simulink model "Model"  (R2021b)
settings: Solver=FixedStepAuto  StartTime=0.0  StopTime=T  FixedStep=0.1  RelTol=1e-3
values from neighbouring files (symbols this model uses):
  A = zeros(length(w_0))    [Model_script.m]
  a = R_E + 550    [Model_script.m]    (also in Orbit_Model.m)
  A0 = eye(3)    [Model_script.m]
  actuators_matrix = [1 0 0; 0 1 0; 0 0 1]    [Model_script.m]
  alpha = deg2rad(11.5)    [Model_script.m]
  Area_mb = diag([A1 A2 A3 A4 A5 A6])    [Model_script.m]
  Area_sp = diag([A7 A8 A9 A10])    [Model_script.m]
  around_boresight = deg2rad(dms2degrees([0,0,around_boresight]))    [Model_script.m]
  B = diag([1/Ix, 1/Iy, 1/Iz])    [Model_script.m]
  cross_boresight = deg2rad(dms2degrees([0,0,cross_boresight]))    [Model_script.m]
  e = 0.0001824    [Model_script.m]    (also in Orbit_Model.m)
  epsilon = deg2rad(23.45)    [Model_script.m]
  H0 = ( g1_0^2 + g1_1^2 + h1_1^2 )^(1/2)    (= 3.0115258674e-05)    [Model_script.m]
  h_N_target = [0; 0; I(3,3)*n]    [Model_script.m]
  I = I_mb + I_depl    [Model_script.m]
  i = deg2rad(53.0545)    [Model_script.m]    (also in Orbit_Model.m)
  I_inv = inv(I)    [Model_script.m]
  i_matrix = [1 0 0; 0 cos(i) sin(i); 0 -sin(i) cos(i)]    [Model_script.m]
  Kb = 1e10    (= 10000000000)    [Model_script.m]
  Kd = 5*1e-4*ones(length(w_0),1)    [Model_script.m]
  Kp = 5*1e-3*ones(length(w_0),1)    [Model_script.m]
  m = [0.01; 0.05; 0.01]    [Model_script.m]
  m_N_unit = zeros(size(m_N,1),size(m_N,2))    [Model_script.m]
  mu_E = astroConstants(13)    [Model_script.m]    (also in Orbit_Model.m)
  n = sqrt(mu_E/(a^3))    [Model_script.m]    (also in Orbit_Model.m)
  n4 = -n1    [Model_script.m]
  N_b_mb = [n1'; n2'; n3'; n4'; n5'; n6']    [Model_script.m]
  N_b_sp = [n7'; n8'; n9'; n10']    [Model_script.m]
  n_sun = 2*pi/T_sun    (= 1.99238499086e-07)    [Model_script.m]
  P = Fe/c    (= 4.52666666667e-06)    [Model_script.m]
  Q = zeros(length(w_0))    [Model_script.m]
  R = zeros(length(w_0))    [Model_script.m]
  R_E = astroConstants(23)    [Model_script.m]    (also in Orbit_Model.m)
  r_mb = [base/2 0 0; 0 base/2 0; 0 0 height/2; -base/2 0 0; 0 -base/2 0; 0 0 -height/2]    [Model_script.m]
  r_sp = [0 length_p1/2+base/2 0; 0 length_p1/2+base/2 0; 0 -length_p2/2-base/2 0; 0 -length_p2/2-base/2 0]    [Model_script.m]
  rho_s_mb = 0.3    [Model_script.m]
  rho_s_sp = 0    [Model_script.m]
  Rs = astroConstants(2)    [Model_script.m]
  star_sensor_tolerance = deg2rad(star_sensor_tolerance)    [Model_script.m]
  theta0 = deg2rad(0)    [Model_script.m]    (also in Orbit_Model.m)
  unit = [1 0 0]'    [Model_script.m]
  v1 = [0 1 -1]'    [Model_script.m]
  v2 = [-1 0 1]'    [Model_script.m]
  v3 = [1 -1 0]'    [Model_script.m]
  w_0 = [wx_0 wy_0 wz_0]'    [Model_script.m]
  w_E = deg2rad(15.04)/3600    [Model_script.m]    (also in Orbit_Model.m = deg2rad(15.04/3600))
  w_target = [0; 0; n]    [Model_script.m]
  weight = 1/6    (= 0.166666666667)    [Model_script.m]
  wy_0 = 0.7    [Model_script.m]
undefined symbols (not defined in the file or in its folder): phi0, psi0, q0
libraries: matrix_library x15, vrlib x12, dspmtrx3 x3, sharedutil x2
(part 2 of 2)

== system Model/Environment/GG Torque/Gravity Gradient ==
  A_BL : Inport
  R_orbit : Inport  Port=2
  Constant4 : Constant  Value=I
  Cross Product1 : matrix_library/Cross Product
      settings: SourceProductBaseCode=SL
  MatrixMultiply4 : Product  Multiplication=Matrix(*)
  Product : Product
  To Workspace : ToWorkspace  VariableName=c_vector  SampleTime=-1
  creation of coefficient 3*mu_E/(R^3) : Subsystem
  creation of vector c : Subsystem
  T_GG : Outport
  wires:
  Constant4/1 -> MatrixMultiply4/1
  MatrixMultiply4/1 -> Cross Product1/2
  Cross Product1/1 -> Product/2
  Product/1 -> T_GG/1
  creation of vector c/1(c) -> To Workspace/1, MatrixMultiply4/2, Cross Product1/1
  A_BL/1 -> creation of vector c/1(A_BL)
  R_orbit/1 -> creation of coefficient 3*mu_E/(R^3)/1(In1)
  creation of coefficient 3*mu_E/(R^3)/1(Out1) -> Product/1

== system Model/Environment/GG Torque/Transformation from A_B//N to A_B//L ==
  A_B/N : Inport
  theta : Inport  Port=2
  Constant : Constant  Value=i_matrix
  Matrix Multiply : Product  Multiplication=Matrix(*)
  MatrixMultiply1 : Product  Multiplication=Matrix(*)
  Transpose : Math  Operator=transpose  SaturateOnIntegerOverflow=on
  creation of A L/N : Subsystem
  A_B/L : Outport
  wires:
  A_B/N/1 -> MatrixMultiply1/1
  Transpose/1 -> MatrixMultiply1/2
  MatrixMultiply1/1 -> A_B/L/1  "A_BL"
  creation of A L/N/1(A_L/N) -> Matrix Multiply/1
  Constant/1 -> Matrix Multiply/2
  Matrix Multiply/1 -> Transpose/1
  theta/1 -> creation of A L/N/1(theta)

== system Model/Environment/Magnetic Torque/magnetic field of Earth (modelled as dipole) in body frame ==
  A_B/N : Inport
  r_N : Inport  Port=2
  Matrix Multiply : Product  Multiplication=Matrix(*)
  b_N : Subsystem
  b_B : Outport
  wires:
  b_N/1(b_N) -> Matrix Multiply/2
  r_N/1 -> b_N/1(r_N)
  A_B/N/1 -> Matrix Multiply/1
  Matrix Multiply/1 -> b_B/1

== system Model/Environment/SRP Torque/SRP Force on spacecraft main body ==
  S_B : Inport
  (1-rho_s)*Sb : Subsystem
  (2*rho_s*cos(theta)+2/3*rho_d)*Nb : Subsystem
  -PA*cos(theta) : Subsystem
  MatrixMultiply3 : Product  Multiplication=Matrix(*)
  Sum2 : Sum  Inputs=|++
  Switch to compute only force of exposed surfaces : Subsystem  TreatAsAtomicUnit=on
  compiute angle between incoming radiation and surface : Subsystem
  F_mb : Outport
  wires:
  S_B/1 -> (1-rho_s)*Sb/1(In1), compiute angle between incoming radiation and surface/1(S_B)
  compiute angle between incoming radiation and surface/1(cos_theta_mb) -> Switch to compute only force of exposed surfaces/1(In1)
  -PA*cos(theta)/1(Out1) -> MatrixMultiply3/1
  Sum2/1 -> MatrixMultiply3/2
  (1-rho_s)*Sb/1(Out1) -> Sum2/1
  (2*rho_s*cos(theta)+2/3*rho_d)*Nb/1(Out1) -> Sum2/2
  MatrixMultiply3/1 -> F_mb/1
  Switch to compute only force of exposed surfaces/1(Out1) -> -PA*cos(theta)/1(Input), (2*rho_s*cos(theta)+2/3*rho_d)*Nb/1(In1)

== system Model/Environment/SRP Torque/SRP Force on spacecraft solar panels ==
  S_B : Inport
  (1-rho_s)*Sb : Subsystem
  (2*rho_s*cos(theta)+2/3*rho_d)*Nb : Subsystem
  -PA*cos(theta) : Subsystem
  MatrixMultiply3 : Product  Multiplication=Matrix(*)
  Sum2 : Sum  Inputs=|++
  Switch to compute only force of exposed surfaces : Subsystem  TreatAsAtomicUnit=on
  compiute angle between incoming radiation and surface : Subsystem
  F_sp : Outport
  wires:
  S_B/1 -> (1-rho_s)*Sb/1(In1), compiute angle between incoming radiation and surface/1(S_B)
  compiute angle between incoming radiation and surface/1(cos_theta_sp) -> Switch to compute only force of exposed surfaces/1(In1)
  -PA*cos(theta)/1(Out1) -> MatrixMultiply3/1
  Sum2/1 -> MatrixMultiply3/2
  (1-rho_s)*Sb/1(Out1) -> Sum2/1
  (2*rho_s*cos(theta)+2/3*rho_d)*Nb/1(Out1) -> Sum2/2
  MatrixMultiply3/1 -> F_sp/1
  Switch to compute only force of exposed surfaces/1(Out1) -> (2*rho_s*cos(theta)+2/3*rho_d)*Nb/1(In1), -PA*cos(theta)/1(In1)

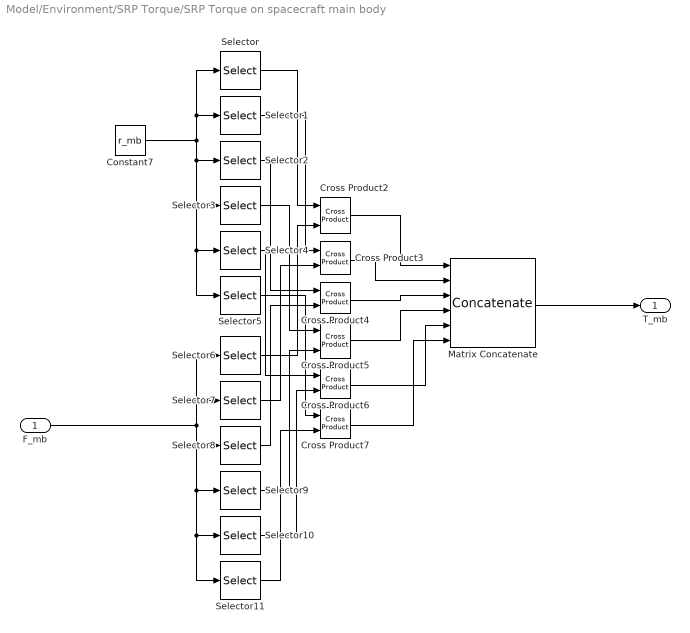
== system Model/Environment/SRP Torque/SRP Torque on spacecraft main body ==
  F_mb : Inport
  Constant7 : Constant  Value=r_mb
  Cross Product{2..7} (6 alike) : matrix_library/Cross Product
      settings: SourceProductBaseCode=SL
  Matrix Concatenate : Concatenate  NumInputs=6  Mode=Multidimensional array
  Selector : Selector  NumberOfDimensions=2  InputPortWidth=3  IndexOptions=Starting index (dialog),Starting index (dialog)  Indices=1,1  OutputSizes=1,3
  Selector1 : Selector  NumberOfDimensions=2  InputPortWidth=3  IndexOptions=Starting index (dialog),Starting index (dialog)  Indices=2,1  OutputSizes=1,3
  Selector10 : Selector  NumberOfDimensions=2  InputPortWidth=3  IndexOptions=Starting index (dialog),Starting index (dialog)  Indices=5,1  OutputSizes=1,3
  Selector11 : Selector  NumberOfDimensions=2  InputPortWidth=3  IndexOptions=Starting index (dialog),Starting index (dialog)  Indices=6,1  OutputSizes=1,3
  Selector2 : Selector  NumberOfDimensions=2  InputPortWidth=3  IndexOptions=Starting index (dialog),Starting index (dialog)  Indices=3,1  OutputSizes=1,3
  Selector3 : Selector  NumberOfDimensions=2  InputPortWidth=3  IndexOptions=Starting index (dialog),Starting index (dialog)  Indices=4,1  OutputSizes=1,3
  Selector4 : Selector  NumberOfDimensions=2  InputPortWidth=3  IndexOptions=Starting index (dialog),Starting index (dialog)  Indices=5,1  OutputSizes=1,3
  Selector5 : Selector  NumberOfDimensions=2  InputPortWidth=3  IndexOptions=Starting index (dialog),Starting index (dialog)  Indices=6,1  OutputSizes=1,3
  Selector6 : Selector  NumberOfDimensions=2  InputPortWidth=3  IndexOptions=Starting index (dialog),Starting index (dialog)  Indices=1,1  OutputSizes=1,3
  Selector7 : Selector  NumberOfDimensions=2  InputPortWidth=3  IndexOptions=Starting index (dialog),Starting index (dialog)  Indices=2,1  OutputSizes=1,3
  Selector8 : Selector  NumberOfDimensions=2  InputPortWidth=3  IndexOptions=Starting index (dialog),Starting index (dialog)  Indices=3,1  OutputSizes=1,3
  Selector9 : Selector  NumberOfDimensions=2  InputPortWidth=3  IndexOptions=Starting index (dialog),Starting index (dialog)  Indices=4,1  OutputSizes=1,3
  T_mb : Outport
  wires:
  Constant7/1 -> Selector2/1, Selector5/1, Selector4/1, Selector3/1, Selector1/1, Selector/1
  Selector5/1 -> Cross Product7/1
  Selector10/1 -> Cross Product6/2
  Selector/1 -> Cross Product2/1
  F_mb/1 -> Selector8/1, Selector11/1, Selector10/1, Selector9/1, Selector7/1, Selector6/1
  Matrix Concatenate/1 -> T_mb/1
  Selector7/1 -> Cross Product3/2
  Cross Product3/1 -> Matrix Concatenate/2
  Selector2/1 -> Cross Product4/1
  Selector9/1 -> Cross Product5/2
  Cross Product6/1 -> Matrix Concatenate/5
  Selector6/1 -> Cross Product2/2
  Selector1/1 -> Cross Product3/1
  Cross Product2/1 -> Matrix Concatenate/1
  Selector11/1 -> Cross Product7/2
  Cross Product5/1 -> Matrix Concatenate/4
  Selector4/1 -> Cross Product6/1
  Selector3/1 -> Cross Product5/1
  Cross Product4/1 -> Matrix Concatenate/3
  Cross Product7/1 -> Matrix Concatenate/6
  Selector8/1 -> Cross Product4/2

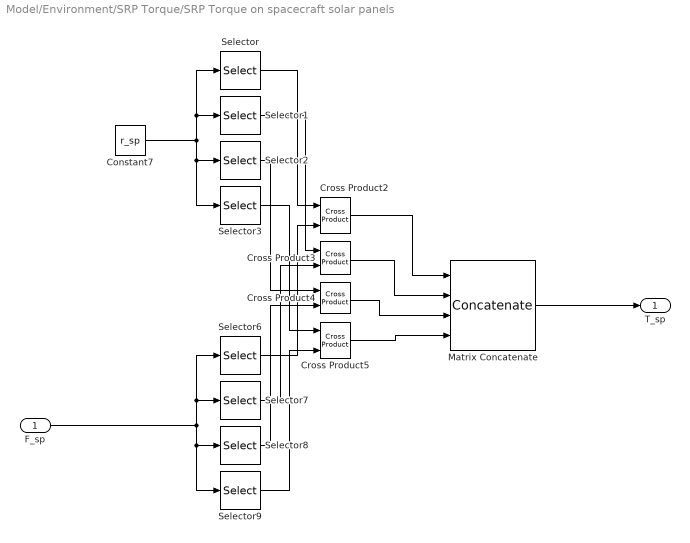
== system Model/Environment/SRP Torque/SRP Torque on spacecraft solar panels ==
  F_sp : Inport
  Constant7 : Constant  Value=r_sp
  Cross Product{2..5} (4 alike) : matrix_library/Cross Product
      settings: SourceProductBaseCode=SL
  Matrix Concatenate : Concatenate  NumInputs=4  Mode=Multidimensional array
  Selector : Selector  NumberOfDimensions=2  InputPortWidth=3  IndexOptions=Starting index (dialog),Starting index (dialog)  Indices=1,1  OutputSizes=1,3
  Selector1 : Selector  NumberOfDimensions=2  InputPortWidth=3  IndexOptions=Starting index (dialog),Starting index (dialog)  Indices=2,1  OutputSizes=1,3
  Selector2 : Selector  NumberOfDimensions=2  InputPortWidth=3  IndexOptions=Starting index (dialog),Starting index (dialog)  Indices=3,1  OutputSizes=1,3
  Selector3 : Selector  NumberOfDimensions=2  InputPortWidth=3  IndexOptions=Starting index (dialog),Starting index (dialog)  Indices=4,1  OutputSizes=1,3
  Selector6 : Selector  NumberOfDimensions=2  InputPortWidth=3  IndexOptions=Starting index (dialog),Starting index (dialog)  Indices=1,1  OutputSizes=1,3
  Selector7 : Selector  NumberOfDimensions=2  InputPortWidth=3  IndexOptions=Starting index (dialog),Starting index (dialog)  Indices=2,1  OutputSizes=1,3
  Selector8 : Selector  NumberOfDimensions=2  InputPortWidth=3  IndexOptions=Starting index (dialog),Starting index (dialog)  Indices=3,1  OutputSizes=1,3
  Selector9 : Selector  NumberOfDimensions=2  InputPortWidth=3  IndexOptions=Starting index (dialog),Starting index (dialog)  Indices=4,1  OutputSizes=1,3
  T_sp : Outport
  wires:
  Constant7/1 -> Selector2/1, Selector3/1, Selector1/1, Selector/1
  Selector/1 -> Cross Product2/1
  F_sp/1 -> Selector8/1, Selector9/1, Selector7/1, Selector6/1
  Matrix Concatenate/1 -> T_sp/1
  Selector7/1 -> Cross Product3/2
  Cross Product3/1 -> Matrix Concatenate/2
  Selector2/1 -> Cross Product4/1
  Selector9/1 -> Cross Product5/2
  Selector6/1 -> Cross Product2/2
  Selector1/1 -> Cross Product3/1
  Cross Product2/1 -> Matrix Concatenate/1
  Cross Product5/1 -> Matrix Concatenate/4
  Selector3/1 -> Cross Product5/1
  Cross Product4/1 -> Matrix Concatenate/3
  Selector8/1 -> Cross Product4/2

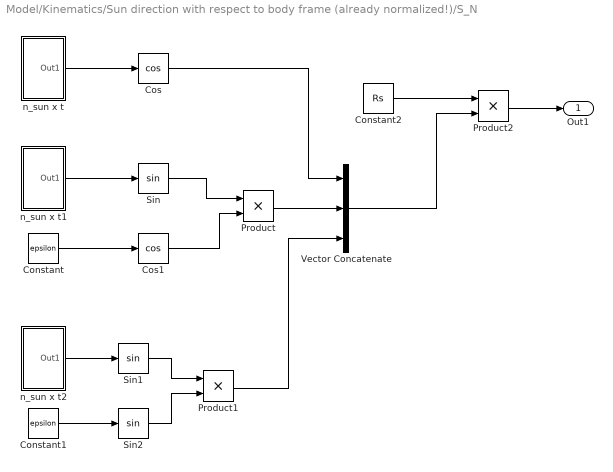
== system Model/Kinematics/Sun direction with respect to body frame (already normalized!)/S_N ==
  Constant : Constant  Value=epsilon
  Constant1 : Constant  Value=epsilon
  Constant2 : Constant  Value=Rs
  Cos : Trigonometry  Operator=cos
  Cos1 : Trigonometry  Operator=cos
  Product : Product
  Product1 : Product
  Product2 : Product
  Sin : Trigonometry
  Sin1 : Trigonometry
  Sin2 : Trigonometry
  Vector Concatenate : Concatenate  NumInputs=3
  n_sun x t : Subsystem
  n_sun x t1 : Subsystem
  n_sun x t2 : Subsystem
  Out1 : Outport
  wires:
  n_sun x t2/1(Out1) -> Sin1/1
  Vector Concatenate/1 -> Product2/2
  Sin2/1 -> Product1/2
  Sin/1 -> Product/1
  n_sun x t1/1(Out1) -> Sin/1
  Product1/1 -> Vector Concatenate/3
  Constant2/1 -> Product2/1
  Cos/1 -> Vector Concatenate/1
  Cos1/1 -> Product/2
  Product/1 -> Vector Concatenate/2
  n_sun x t/1(Out1) -> Cos/1
  Constant1/1 -> Sin2/1
  Sin1/1 -> Product1/1
  Constant/1 -> Cos1/1
  Product2/1 -> Out1/1

== system Model/Kinematics/radius of orbit in body frame and transformation matrix from inertial frame to body frame /finder of A_B//N(t) ==
  w : Inport
  Demux : Demux  Outputs=3
  Gain : Gain  Gain=-1
  Integrator1 : Integrator  InitialCondition=A0
  MatrixMultiply : Product  Multiplication=Matrix(*)
  w_hat : Subsystem
  A(t) : Outport
  wires:
  w/1 -> Demux/1
  Gain/1 -> MatrixMultiply/1
  Integrator1/1 -> A(t)/1, MatrixMultiply/2  "A(t)"
  w_hat/1(Out1) -> Gain/1
  Demux/3 -> w_hat/3(w_z)  "w_z"
  Demux/2 -> w_hat/2(w_y)  "w_y"
  Demux/1 -> w_hat/1(w_x)  "w_x"
  MatrixMultiply/1 -> Integrator1/1

== system Model/Kinematics/radius of orbit in body frame and transformation matrix from inertial frame to body frame /orthonormalization of matrix A(t) ==
  A(t) : Inport
  Gain7 : Gain  Gain=3/2
  Gain8 : Gain  Gain=1/2
  MatrixMultiply3 : Product  Multiplication=Matrix(*)
  MatrixMultiply4 : Product  Multiplication=Matrix(*)
  Sum : Sum  Inputs=+-
  Transpose : Math  Operator=transpose  SaturateOnIntegerOverflow=on
  A_orthonorm : Outport
  wires:
  Transpose/1 -> MatrixMultiply3/2
  MatrixMultiply4/1 -> Sum/2
  MatrixMultiply3/1 -> MatrixMultiply4/1
  Gain7/1 -> Sum/1
  Gain8/1 -> MatrixMultiply4/2  "A/2"
  A(t)/1 -> Gain8/1, Transpose/1, MatrixMultiply3/1, Gain7/1
  Sum/1 -> A_orthonorm/1  "A_orthonorm"

== system Model/Kinematics/radius of orbit in body frame and transformation matrix from inertial frame to body frame /radius of orbit in the inertial reference frame ==
  Product2 : Product
  Radius of orbit : Subsystem
  Theta : Subsystem
  vector [cos(theta); sin(theta)cos(i); sin(theta)sin(i)] : Subsystem
  theta : Outport
  r_N : Outport  Port=2
  R_orbit : Outport  Port=3
  wires:
  Theta/1(theta) -> vector [cos(theta); sin(theta)cos(i); sin(theta)sin(i)]/1(In1), theta/1, Radius of orbit/1(theta)
  Radius of orbit/1(R_orbit) -> Product2/1, R_orbit/1
  Product2/1 -> r_N/1
  vector [cos(theta); sin(theta)cos(i); sin(theta)sin(i)]/1(Out1) -> Product2/2

== system Model/Pointing error/pointing error evaluated in inertial frame/Pointing error ==
  h_N : Inport
  Abs : Abs
  Constant : Constant  Value=h_N_target  VectorParams1D=off
  Sum : Sum  Inputs=+-
  err : Outport
  wires:
  Constant/1 -> Sum/2
  h_N/1 -> Sum/1
  Sum/1 -> Abs/1
  Abs/1 -> err/1

== system Model/Pointing error/pointing error evaluated in inertial frame/angular momentum in inertial frame ==
  A_B/N : Inport
  h_B : Inport  Port=2
  Matrix Multiply : Product  Multiplication=Matrix(*)
  Transpose : Math  Operator=transpose  SaturateOnIntegerOverflow=on
  h_N : Outport
  wires:
  Transpose/1 -> Matrix Multiply/1
  Matrix Multiply/1 -> h_N/1
  A_B/N/1 -> Transpose/1
  h_B/1 -> Matrix Multiply/2

== system Model/Subsystem1/w_hat/Subsystem ==
  w_x : Inport
  w_y : Inport  Port=2
  w_z : Inport  Port=3
  Constant2 : Constant  Value=v1
  Product2 : Product
  Vector Concatenate : Concatenate  NumInputs=3
  Out1 : Outport
  wires:
  Product2/1 -> Out1/1
  Vector Concatenate/1 -> Product2/1
  Constant2/1 -> Product2/2
  w_x/1 -> Vector Concatenate/1
  w_z/1 -> Vector Concatenate/2
  w_y/1 -> Vector Concatenate/3

== system Model/Subsystem1/w_hat/Subsystem1 ==
  w_x : Inport
  w_y : Inport  Port=2
  w_z : Inport  Port=3
  Constant4 : Constant  Value=v2
  Product4 : Product
  Vector Concatenate2 : Concatenate  NumInputs=3
  Out1 : Outport
  wires:
  Constant4/1 -> Product4/2
  Vector Concatenate2/1 -> Product4/1
  Product4/1 -> Out1/1
  w_x/1 -> Vector Concatenate2/3
  w_y/1 -> Vector Concatenate2/2
  w_z/1 -> Vector Concatenate2/1

== system Model/Subsystem1/w_hat/Subsystem2 ==
  w_x : Inport
  w_y : Inport  Port=2
  w_z : Inport  Port=3
  Constant3 : Constant  Value=v3
  Product3 : Product
  Vector Concatenate1 : Concatenate  NumInputs=3
  Out1 : Outport
  wires:
  Product3/1 -> Out1/1
  Constant3/1 -> Product3/2
  w_y/1 -> Vector Concatenate1/1
  Vector Concatenate1/1 -> Product3/1
  w_x/1 -> Vector Concatenate1/2
  w_z/1 -> Vector Concatenate1/3

== system Model/Environment/GG Torque/Gravity Gradient/creation of coefficient 3*mu_E//(R^3) ==
  In1 : Inport
  Constant : Constant  Value=3
  Constant1 : Constant  Value=mu_E
  Divide : Product  Inputs=*/
  Gain : Gain  Gain=3
  Power : Math  Operator=pow  SaturateOnIntegerOverflow=on
  Out1 : Outport
  wires:
  Divide/1 -> Out1/1
  Power/1 -> Divide/2
  Constant/1 -> Power/2
  In1/1 -> Power/1
  Constant1/1 -> Gain/1
  Gain/1 -> Divide/1

== system Model/Environment/GG Torque/Gravity Gradient/creation of vector c ==
  A_BL : Inport
  Constant : Constant  Value=unit  VectorParams1D=off
  MatrixMultiply3 : Product  Multiplication=Matrix(*)
  c : Outport
  wires:
  A_BL/1 -> MatrixMultiply3/1
  MatrixMultiply3/1 -> c/1
  Constant/1 -> MatrixMultiply3/2

== system Model/Environment/GG Torque/Transformation from A_B//N to A_B//L/creation of A L//N ==
  theta : Inport
  Matrix Concatenate : Concatenate  NumInputs=3  Mode=Multidimensional array  ConcatenateDimension=2
  first column of A_L/N : Subsystem
  second column of A_L/N : Subsystem
  third column of A_L/N : Subsystem
  A_L/N : Outport
  wires:
  second column of A_L/N/1(A_L/N (:,2)) -> Matrix Concatenate/2
  Matrix Concatenate/1 -> A_L/N/1
  first column of A_L/N/1(A_L/N (:,1)) -> Matrix Concatenate/1
  third column of A_L/N/1(A_L/N (:,3)) -> Matrix Concatenate/3
  theta/1 -> second column of A_L/N/1(theta), first column of A_L/N/1(theta)

== system Model/Environment/Magnetic Torque/magnetic field of Earth (modelled as dipole) in body frame/b_N ==
  r_N : Inport
  Product : Product
  R^3*H0/(r^3) : Subsystem
  "[3*(m_unit*r_unit)*r_unit - m_unit)" : Subsystem
  magnetic unit vector of Earth : Subsystem
  normalization of r_N : Subsystem
  b_N : Outport
  wires:
  magnetic unit vector of Earth/1(Out1) -> "[3*(m_unit*r_unit)*r_unit - m_unit)"/1(m_unit)
  normalization of r_N/1(normalized r_N) -> "[3*(m_unit*r_unit)*r_unit - m_unit)"/2(normalized r_N)
  normalization of r_N/2(norm(r_N)) -> R^3*H0/(r^3)/1(normalized r_N)
  "[3*(m_unit*r_unit)*r_unit - m_unit)"/1(Out1) -> Product/1
  Product/1 -> b_N/1
  R^3*H0/(r^3)/1(coeff) -> Product/2
  r_N/1 -> normalization of r_N/1(r_N)

== system Model/Environment/SRP Torque/SRP Force on spacecraft main body/(1-rho_s)*Sb ==
  In1 : Inport
  Constant2 : Constant
  Constant3 : Constant  Value=rho_s_mb
  Product1 : Product
  Sum : Sum  Inputs=+-
  Transpose1 : Math  Operator=transpose  SaturateOnIntegerOverflow=on
  Out1 : Outport
  wires:
  Constant2/1 -> Sum/1
  Sum/1 -> Product1/1
  Transpose1/1 -> Product1/2
  Product1/1 -> Out1/1
  Constant3/1 -> Sum/2
  In1/1 -> Transpose1/1

== system Model/Environment/SRP Torque/SRP Force on spacecraft main body/(2*rho_s*cos(theta)+2//3*rho_d)*Nb ==
  In1 : Inport
  Constant1 : Constant  Value=rho_s_mb
  Constant2 : Constant  Value=ones(6,1)
  Constant4 : Constant  Value=rho_s_mb
  Constant6 : Constant  Value=N_b_mb
  Gain1 : Gain  Gain=2
  Gain2 : Gain  Gain=2/3
  MatrixMultiply2 : Product  Multiplication=Matrix(*)
  Product : Product
  Product2 : Product
  Sum1 : Sum  Inputs=|++
  Out1 : Outport
  wires:
  Gain2/1 -> Product/1
  Product/1 -> Sum1/1
  MatrixMultiply2/1 -> Out1/1
  Constant4/1 -> Gain1/1
  In1/1 -> Product2/2
  Constant6/1 -> MatrixMultiply2/2
  Gain1/1 -> Product2/1
  Product2/1 -> Sum1/2
  Sum1/1 -> MatrixMultiply2/1
  Constant1/1 -> Gain2/1
  Constant2/1 -> Product/2

== system Model/Environment/SRP Torque/SRP Force on spacecraft main body/-PA*cos(theta) ==
  Input : Inport
  Constant1 : Constant  Value=Area_mb
  Gain : Gain  Gain=-P
  Matrix Multiply : Product  Multiplication=Matrix(*)
  Out1 : Outport
  wires:
  Matrix Multiply/1 -> Out1/1
  Gain/1 -> Matrix Multiply/1
  Constant1/1 -> Gain/1
  Input/1 -> Matrix Multiply/2

== system Model/Environment/SRP Torque/SRP Force on spacecraft main body/Switch to compute only force of exposed surfaces ==
  In1 : Inport  Partition=on  PartitionDimension=1  PartitionWidth=1  PartitionOffset=0
  Constant : Constant  Value=0
  For Each : ForEach  DisableCoverage=on
  Switch : Switch  Criteria=u2 > Threshold
  Out1 : Outport  ConcatenationDimension=1
  wires:
  In1/1 -> Switch/1, Switch/2
  Constant/1 -> Switch/3
  Switch/1 -> Out1/1

== system Model/Environment/SRP Torque/SRP Force on spacecraft main body/compiute angle between incoming radiation and surface ==
  S_B : Inport
  Constant : Constant  Value=N_b_mb
  MatrixMultiply : Product  Multiplication=Matrix(*)
  cos_theta_mb : Outport
  wires:
  Constant/1 -> MatrixMultiply/1
  MatrixMultiply/1 -> cos_theta_mb/1
  S_B/1 -> MatrixMultiply/2

== system Model/Environment/SRP Torque/SRP Force on spacecraft solar panels/(1-rho_s)*Sb ==
  In1 : Inport
  Constant2 : Constant
  Constant3 : Constant  Value=rho_s_sp
  Product1 : Product
  Sum : Sum  Inputs=+-
  Transpose1 : Math  Operator=transpose  SaturateOnIntegerOverflow=on
  Out1 : Outport
  wires:
  Constant2/1 -> Sum/1
  Sum/1 -> Product1/1
  Transpose1/1 -> Product1/2
  Product1/1 -> Out1/1
  Constant3/1 -> Sum/2
  In1/1 -> Transpose1/1

== system Model/Environment/SRP Torque/SRP Force on spacecraft solar panels/(2*rho_s*cos(theta)+2//3*rho_d)*Nb ==
  In1 : Inport
  Constant1 : Constant  Value=rho_s_sp
  Constant2 : Constant  Value=ones(4,1)
  Constant4 : Constant  Value=rho_s_sp
  Constant6 : Constant  Value=N_b_sp
  Gain1 : Gain  Gain=2
  Gain2 : Gain  Gain=2/3
  MatrixMultiply2 : Product  Multiplication=Matrix(*)
  Product : Product
  Product2 : Product
  Sum1 : Sum  Inputs=|++
  Out1 : Outport
  wires:
  Gain2/1 -> Product/1
  Product/1 -> Sum1/1
  MatrixMultiply2/1 -> Out1/1
  Constant4/1 -> Gain1/1
  In1/1 -> Product2/2
  Constant6/1 -> MatrixMultiply2/2
  Gain1/1 -> Product2/1
  Product2/1 -> Sum1/2
  Sum1/1 -> MatrixMultiply2/1
  Constant1/1 -> Gain2/1
  Constant2/1 -> Product/2

== system Model/Environment/SRP Torque/SRP Force on spacecraft solar panels/-PA*cos(theta) ==
  In1 : Inport
  Constant1 : Constant  Value=Area_sp
  Gain : Gain  Gain=-P
  MatrixMultiply : Product  Multiplication=Matrix(*)
  Out1 : Outport
  wires:
  Constant1/1 -> Gain/1
  Gain/1 -> MatrixMultiply/1
  MatrixMultiply/1 -> Out1/1
  In1/1 -> MatrixMultiply/2

== system Model/Environment/SRP Torque/SRP Force on spacecraft solar panels/Switch to compute only force of exposed surfaces ==
  In1 : Inport  Partition=on  PartitionDimension=1  PartitionWidth=1  PartitionOffset=0
  Constant : Constant  Value=0
  For Each : ForEach  DisableCoverage=on
  Switch : Switch  Criteria=u2 > Threshold
  Out1 : Outport  ConcatenationDimension=1
  wires:
  In1/1 -> Switch/1, Switch/2
  Constant/1 -> Switch/3
  Switch/1 -> Out1/1

== system Model/Environment/SRP Torque/SRP Force on spacecraft solar panels/compiute angle between incoming radiation and surface ==
  S_B : Inport
  Constant : Constant  Value=N_b_sp
  MatrixMultiply : Product  Multiplication=Matrix(*)
  cos_theta_sp : Outport
  wires:
  Constant/1 -> MatrixMultiply/1
  MatrixMultiply/1 -> cos_theta_sp/1
  S_B/1 -> MatrixMultiply/2

== system Model/Kinematics/Sun direction with respect to body frame (already normalized!)/S_N/n_sun x t ==
  Clock : Clock
  Constant : Constant  Value=n_sun
  Product : Product
  Out1 : Outport
  wires:
  Constant/1 -> Product/1
  Clock/1 -> Product/2
  Product/1 -> Out1/1

== system Model/Kinematics/Sun direction with respect to body frame (already normalized!)/S_N/n_sun x t1 ==
  Clock : Clock
  Constant : Constant  Value=n_sun
  Product : Product
  Out1 : Outport
  wires:
  Product/1 -> Out1/1
  Clock/1 -> Product/2
  Constant/1 -> Product/1

== system Model/Kinematics/Sun direction with respect to body frame (already normalized!)/S_N/n_sun x t2 ==
  Clock : Clock
  Constant : Constant  Value=n_sun
  Product : Product
  Out1 : Outport
  wires:
  Constant/1 -> Product/1
  Clock/1 -> Product/2
  Product/1 -> Out1/1

== system Model/Kinematics/radius of orbit in body frame and transformation matrix from inertial frame to body frame /finder of A_B//N(t)/w_hat ==
  w_x : Inport
  w_y : Inport  Port=2
  w_z : Inport  Port=3
  Matrix Concatenate : Concatenate  NumInputs=3  Mode=Multidimensional array  ConcatenateDimension=2
  Scope : Scope  NumInputPorts=3
  Subsystem : Subsystem
  Subsystem1 : Subsystem
  Subsystem2 : Subsystem
  Out1 : Outport
  wires:
  w_y/1 -> Subsystem1/2(w_y), Subsystem/2(w_y), Subsystem2/2(w_y), Scope/2
  w_z/1 -> Subsystem2/3(w_z), Subsystem/3(w_z), Subsystem1/3(w_z), Scope/3
  w_x/1 -> Subsystem2/1(w_x), Subsystem/1(w_x), Subsystem1/1(w_x), Scope/1
  Subsystem2/1(Out1) -> Matrix Concatenate/3
  Subsystem1/1(Out1) -> Matrix Concatenate/2
  Subsystem/1(Out1) -> Matrix Concatenate/1
  Matrix Concatenate/1 -> Out1/1

== system Model/Kinematics/radius of orbit in body frame and transformation matrix from inertial frame to body frame /radius of orbit in the inertial reference frame/Radius of orbit ==
  theta : Inport
  Constant : Constant  Value=a
  Constant1 : Constant
  Constant2 : Constant  Value=e
  Constant3 : Constant
  Constant4 : Constant  Value=e
  Cos : Trigonometry  Operator=cos
  Divide : Product  Inputs=*/
  Product : Product
  Product1 : Product
  Square1 : Math  Operator=square  SaturateOnIntegerOverflow=on
  Sum : Sum  Inputs=|++
  Sum1 : Sum  Inputs=|+-
  R_orbit : Outport
  wires:
  Sum/1 -> Divide/2
  Constant1/1 -> Sum/1
  Square1/1 -> Sum1/2
  Product1/1 -> Sum/2
  Constant2/1 -> Product1/1
  Constant/1 -> Product/2
  Divide/1 -> R_orbit/1
  Cos/1 -> Product1/2
  Sum1/1 -> Product/1
  theta/1 -> Cos/1
  Constant4/1 -> Square1/1
  Constant3/1 -> Sum1/1
  Product/1 -> Divide/1

== system Model/Kinematics/radius of orbit in body frame and transformation matrix from inertial frame to body frame /radius of orbit in the inertial reference frame/Theta ==
  Denominator : Subsystem
  Divide : Product  Inputs=*/
  Integrator : Integrator  InitialCondition=theta0
  Numerator : Subsystem
  theta : Outport
  wires:
  Numerator/1(Out1) -> Divide/1
  Denominator/1(Out1) -> Divide/2
  Integrator/1 -> theta/1, Numerator/1(In1)
  Divide/1 -> Integrator/1

== system Model/Kinematics/radius of orbit in body frame and transformation matrix from inertial frame to body frame /radius of orbit in the inertial reference frame/vector [cos(theta); sin(theta)cos(i); sin(theta)sin(i)] ==
  In1 : Inport
  Constant : Constant  Value=i
  Constant1 : Constant  Value=i
  Cos : Trigonometry  Operator=cos
  Cos1 : Trigonometry  Operator=cos
  Product : Product
  Product1 : Product
  Sin : Trigonometry
  Sin1 : Trigonometry
  Sin2 : Trigonometry
  Vector Concatenate : Concatenate  NumInputs=3
  Out1 : Outport
  wires:
  Sin/1 -> Product/1
  Sin2/1 -> Product1/1
  Constant1/1 -> Sin1/1
  Cos/1 -> Vector Concatenate/1
  Product/1 -> Vector Concatenate/2
  In1/1 -> Sin2/1, Sin/1, Cos/1
  Constant/1 -> Cos1/1
  Cos1/1 -> Product/2
  Sin1/1 -> Product1/2
  Product1/1 -> Vector Concatenate/3
  Vector Concatenate/1 -> Out1/1

== system Model/Environment/GG Torque/Transformation from A_B//N to A_B//L/creation of A L//N/first column of A_L//N ==
  theta : Inport
  Constant : Constant  Value=0
  Cos : Trigonometry  Operator=cos
  Gain : Gain  Gain=-1
  Sin : Trigonometry
  Vector Concatenate : Concatenate  NumInputs=3
  A_L/N (:,1) : Outport
  wires:
  Constant/1 -> Vector Concatenate/3
  Cos/1 -> Vector Concatenate/1
  Vector Concatenate/1 -> A_L/N (:,1)/1
  Gain/1 -> Vector Concatenate/2
  Sin/1 -> Gain/1
  theta/1 -> Cos/1, Sin/1

== system Model/Environment/GG Torque/Transformation from A_B//N to A_B//L/creation of A L//N/second column of A_L//N ==
  theta : Inport
  Constant : Constant  Value=0
  Cos : Trigonometry
  Sin : Trigonometry  Operator=cos
  Vector Concatenate : Concatenate  NumInputs=3
  A_L/N (:,2) : Outport
  wires:
  Constant/1 -> Vector Concatenate/3
  Cos/1 -> Vector Concatenate/1
  Vector Concatenate/1 -> A_L/N (:,2)/1
  Sin/1 -> Vector Concatenate/2
  theta/1 -> Sin/1, Cos/1

== system Model/Environment/GG Torque/Transformation from A_B//N to A_B//L/creation of A L//N/third column of A_L//N ==
  Constant : Constant
  Constant1 : Constant  Value=0
  Constant2 : Constant  Value=0
  Vector Concatenate : Concatenate  NumInputs=3
  A_L/N (:,3) : Outport
  wires:
  Constant/1 -> Vector Concatenate/3
  Vector Concatenate/1 -> A_L/N (:,3)/1
  Constant1/1 -> Vector Concatenate/2
  Constant2/1 -> Vector Concatenate/1

== system Model/Environment/Magnetic Torque/magnetic field of Earth (modelled as dipole) in body frame/b_N/R^3*H0//(r^3) ==
  normalized r_N : Inport
  Constant : Constant  Value=R_E
  Constant1 : Constant  Value=3
  Constant2 : Constant  Value=H0
  Constant3 : Constant  Value=3
  Divide : Product  Inputs=*/
  Power : Math  Operator=pow  SaturateOnIntegerOverflow=on
  Power1 : Math  Operator=pow  SaturateOnIntegerOverflow=on
  Product : Product
  coeff : Outport
  wires:
  Power/1 -> Product/1
  Constant/1 -> Power/1
  Constant2/1 -> Product/2
  Divide/1 -> coeff/1
  Constant1/1 -> Power/2
  Product/1 -> Divide/1
  Constant3/1 -> Power1/2
  normalized r_N/1 -> Power1/1
  Power1/1 -> Divide/2

== system Model/Environment/Magnetic Torque/magnetic field of Earth (modelled as dipole) in body frame/b_N/[3*(m_unit*r_unit)*r_unit - m_unit) ==
  m_unit : Inport
  normalized r_N : Inport  Port=2
  Constant : Constant  Value=3
  Dot Product1 : DotProduct  InputSameDT=on  OutDataTypeStr=Inherit: Inherit via internal rule
  Product : Product
  Product1 : Product
  Sum : Sum  Inputs=-+
  Transpose : Math  Operator=transpose  SaturateOnIntegerOverflow=on
  Out1 : Outport
  wires:
  m_unit/1 -> Dot Product1/1, Sum/1
  Constant/1 -> Product/2
  Dot Product1/1 -> Product/1
  Sum/1 -> Out1/1
  Product/1 -> Product1/1
  normalized r_N/1 -> Product1/2, Dot Product1/2
  Product1/1 -> Transpose/1
  Transpose/1 -> Sum/2

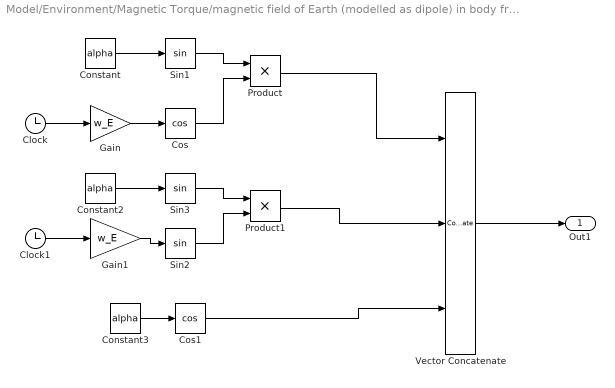
== system Model/Environment/Magnetic Torque/magnetic field of Earth (modelled as dipole) in body frame/b_N/magnetic unit vector of Earth ==
  Clock : Clock
  Clock1 : Clock
  Constant : Constant  Value=alpha
  Constant2 : Constant  Value=alpha
  Constant3 : Constant  Value=alpha
  Cos : Trigonometry  Operator=cos
  Cos1 : Trigonometry  Operator=cos
  Gain : Gain  Gain=w_E
  Gain1 : Gain  Gain=w_E
  Product : Product
  Product1 : Product
  Sin1 : Trigonometry
  Sin2 : Trigonometry
  Sin3 : Trigonometry
  Vector Concatenate : Concatenate  NumInputs=3  Mode=Multidimensional array
  Out1 : Outport
  wires:
  Constant2/1 -> Sin3/1
  Clock/1 -> Gain/1
  Product1/1 -> Vector Concatenate/2
  Sin2/1 -> Product1/2
  Cos1/1 -> Vector Concatenate/3
  Constant/1 -> Sin1/1
  Sin1/1 -> Product/1
  Sin3/1 -> Product1/1
  Gain1/1 -> Sin2/1
  Product/1 -> Vector Concatenate/1
  Constant3/1 -> Cos1/1
  Cos/1 -> Product/2
  Clock1/1 -> Gain1/1
  Gain/1 -> Cos/1
  Vector Concatenate/1 -> Out1/1

== system Model/Environment/Magnetic Torque/magnetic field of Earth (modelled as dipole) in body frame/b_N/normalization of r_N ==
  r_N : Inport
  Divide : Product  Inputs=*/
  norm of r_N : Subsystem
  normalized r_N : Outport
  norm(r_N) : Outport  Port=2
  wires:
  r_N/1 -> Divide/1, norm of r_N/1(In1)
  Divide/1 -> normalized r_N/1
  norm of r_N/1(norm(r_N)) -> norm(r_N)/1, Divide/2

== system Model/Kinematics/radius of orbit in body frame and transformation matrix from inertial frame to body frame /finder of A_B//N(t)/w_hat/Subsystem ==
  w_x : Inport
  w_y : Inport  Port=2
  w_z : Inport  Port=3
  Constant2 : Constant  Value=v1
  Product2 : Product
  Vector Concatenate : Concatenate  NumInputs=3
  Out1 : Outport
  wires:
  Product2/1 -> Out1/1
  Vector Concatenate/1 -> Product2/1
  Constant2/1 -> Product2/2
  w_x/1 -> Vector Concatenate/1
  w_z/1 -> Vector Concatenate/2
  w_y/1 -> Vector Concatenate/3

== system Model/Kinematics/radius of orbit in body frame and transformation matrix from inertial frame to body frame /finder of A_B//N(t)/w_hat/Subsystem1 ==
  w_x : Inport
  w_y : Inport  Port=2
  w_z : Inport  Port=3
  Constant4 : Constant  Value=v2
  Product4 : Product
  Vector Concatenate2 : Concatenate  NumInputs=3
  Out1 : Outport
  wires:
  Constant4/1 -> Product4/2
  Vector Concatenate2/1 -> Product4/1
  Product4/1 -> Out1/1
  w_x/1 -> Vector Concatenate2/3
  w_y/1 -> Vector Concatenate2/2
  w_z/1 -> Vector Concatenate2/1

== system Model/Kinematics/radius of orbit in body frame and transformation matrix from inertial frame to body frame /finder of A_B//N(t)/w_hat/Subsystem2 ==
  w_x : Inport
  w_y : Inport  Port=2
  w_z : Inport  Port=3
  Constant3 : Constant  Value=v3
  Product3 : Product
  Vector Concatenate1 : Concatenate  NumInputs=3
  Out1 : Outport
  wires:
  Product3/1 -> Out1/1
  Constant3/1 -> Product3/2
  w_y/1 -> Vector Concatenate1/1
  Vector Concatenate1/1 -> Product3/1
  w_x/1 -> Vector Concatenate1/2
  w_z/1 -> Vector Concatenate1/3

== system Model/Kinematics/radius of orbit in body frame and transformation matrix from inertial frame to body frame /radius of orbit in the inertial reference frame/Theta/Denominator ==
  Constant3 : Constant
  Constant4 : Constant  Value=e
  Constant5 : Constant  Value=3/2
  Power : Math  Operator=pow  SaturateOnIntegerOverflow=on
  Square1 : Math  Operator=square  SaturateOnIntegerOverflow=on
  Sum1 : Sum  Inputs=|+-
  Out1 : Outport
  wires:
  Constant3/1 -> Sum1/1
  Constant4/1 -> Square1/1
  Sum1/1 -> Power/1
  Square1/1 -> Sum1/2
  Constant5/1 -> Power/2
  Power/1 -> Out1/1

== system Model/Kinematics/radius of orbit in body frame and transformation matrix from inertial frame to body frame /radius of orbit in the inertial reference frame/Theta/Numerator ==
  In1 : Inport
  Constant : Constant  Value=n
  Constant1 : Constant  Value=e
  Constant2 : Constant
  Cos : Trigonometry  Operator=cos
  Product : Product
  Product1 : Product
  Square : Math  Operator=square  SaturateOnIntegerOverflow=on
  Sum : Sum  Inputs=|++
  Out1 : Outport
  wires:
  Constant2/1 -> Sum/2
  Sum/1 -> Square/1
  In1/1 -> Cos/1
  Constant1/1 -> Product/1
  Constant/1 -> Product1/1
  Cos/1 -> Product/2
  Product/1 -> Sum/1
  Square/1 -> Product1/2
  Product1/1 -> Out1/1

== system Model/Environment/Magnetic Torque/magnetic field of Earth (modelled as dipole) in body frame/b_N/normalization of r_N/norm of r_N ==
  In1 : Inport
  Constant1 : Constant  Value=0.5
  Dot Product : DotProduct  InputSameDT=on  OutDataTypeStr=Inherit: Inherit via internal rule
  Power : Math  Operator=pow  SaturateOnIntegerOverflow=on
  norm(r_N) : Outport
  wires:
  In1/1 -> Dot Product/2, Dot Product/1
  Constant1/1 -> Power/2
  Dot Product/1 -> Power/1
  Power/1 -> norm(r_N)/1

== matlab function Model/Attitude Determination (Statistic method)/MATLAB Function ==
  data: U output; u input
function U   =  eigenvector(u)
[U,D]=eig(u);
end

== matlab function Model/Attitude Determination (Statistic method)/MATLAB Function1 ==
  data: u input; V output
function V   =  eigenvector(u)
[V,D]=eig(u);
return

== matlab function Model/Actuators/Pseudoinverse ==
  data: A input; A_pseudoinv output
function A_pseudoinv = fcn(A)

        A_pseudoinv = A'*inv(A*A');

end

== matlab function Model/Control/MATLAB Function ==
  data: A input; B input; K output; Q input; R input; N input; S output; CLP output
function [K,S,CLP] = controller(A,B,Q,R,N)

[K,S,CLP] = lqr(A,B,Q,R,N);

end

== matlab function Model/Control/MATLAB Function1 ==
  data: A_error input; a output
function a  = extraction(A_error)

    ax = A_error(2,3);
    ay = A_error(3,1);
    az = A_error(1,2);
    a = [ax; ay; az];

end

== matlab function Model/Control/MATLAB Function2 ==
  data: a input; Kp input; Kd input; w input; M output; w_target input
function M  = linear_control(a, Kp, Kd, w, w_target)

   M = Kp.*a + Kd.*(w - w_target); 

end
